simulink model "Strujni_nacin"  (R2023b)
settings: Solver=VariableStepAuto  StartTime=0.0  StopTime=stepp.sim_time  RelTol=1e-3
undefined symbols (not defined in the file or in its folder): ccm_m_op, G_sys_ccm, G_sys_dcm, G_Ubat_Ir_DCM, G_Ubat_Ir_full, G_Ubat_Ir_full_m, G_Ubat_Ir_nozero, G_Ubat_Ir_nozero_m, G_Ubat_Ir_red, G_Ubat_Ir_red_m, G_Ubat_Upv_DCM, G_Ubat_Upv_full, G_Ubat_Upv_full_m, G_Ubat_Upv_nozero, G_Ubat_Upv_nozero_m, G_Ubat_Upv_red, G_Ubat_Upv_red_m, G_UPV, G_Upv_IL, Ipv0, Ir, ro_ccm, ro_ccm_m, ro_dcm, stepp, Ubat0_ccm, Upv
settings Model: Creator=teo  LastModifiedBy=teo

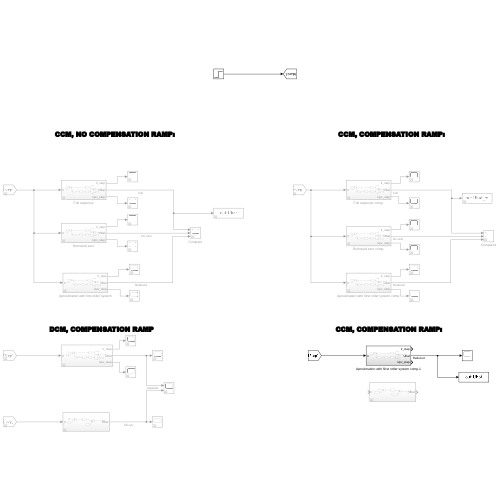
[thumbnail: Simulink's stored preview of the top-level diagram]
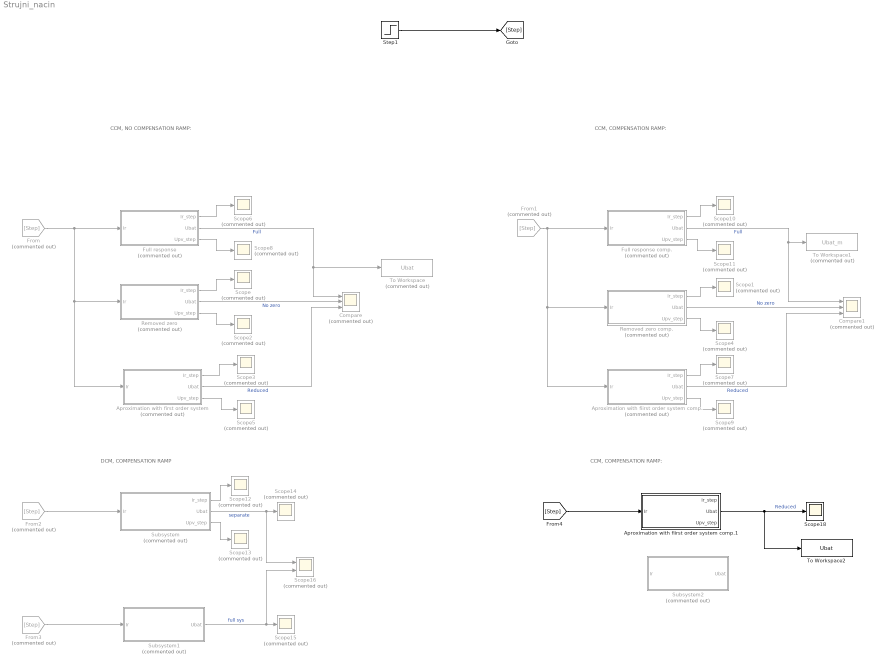
== system Strujni_nacin ==
  note: CCM, NO COMPENSATION RAMP:
  note: CCM, COMPENSATION RAMP:
  note: DCM, COMPENSATION RAMP
  note: CCM, COMPENSATION RAMP:
  Aproximation with fiirst order system comp. : Subsystem  Commented=on
  Aproximation with fiirst order system comp.1 : Subsystem
  Aproximation with first order system : Subsystem  Commented=on
  Compare : Scope  Commented=on  NumInputPorts=3
  Compare1 : Scope  Commented=on  NumInputPorts=3
  From{,1..3} (4 alike) : From  Commented=on  GotoTag=Step
  Full response : Subsystem  Commented=on
  Full response comp. : Subsystem  Commented=on
  Removed zero : Subsystem  Commented=on
  Removed zero comp. : Subsystem  Commented=on
  Scope{,1..15} (16 alike) : Scope  Commented=on
  Scope16 : Scope  Commented=on  NumInputPorts=2
  Scope18 : Scope
  Step1 : Step  Time=stepp.step_time  Before=stepp.ir01  After=stepp.ir02  SampleTime=0
  Subsystem : Subsystem  Commented=on
  Subsystem1 : Subsystem  Commented=on
  Subsystem2 : Subsystem  Commented=on
  To Workspace : ToWorkspace  Commented=on  VariableName=Ubat  SaveFormat=Timeseries  SampleTime=-1
  To Workspace1 : ToWorkspace  Commented=on  VariableName=Ubat_m  SaveFormat=Timeseries  SampleTime=-1
  To Workspace2 : ToWorkspace  VariableName=Ubat  SaveFormat=Timeseries  SampleTime=-1
  wires:
  Step1/1 -> [Step]
  From/1 -> Aproximation with first order system/1(Ir), Removed zero/1(Ir), Full response/1(Ir)
  Full response/1(Ir_step) -> Scope6/1
  Full response/3(Upv_step) -> Scope8/1
  Removed zero/1(Ir_step) -> Scope/1
  Removed zero/3(Upv_step) -> Scope2/1
  Aproximation with first order system/1(Ir_step) -> Scope3/1
  Aproximation with first order system/3(Upv_step) -> Scope5/1
  Removed zero/2(Ubat) -> Compare/2  "No zero"
  Full response/2(Ubat) -> To Workspace/1, Compare/1  "Full"
  Aproximation with first order system/2(Ubat) -> Compare/3  "Reduced"
  Full response comp./3(Upv_step) -> Scope11/1
  Full response comp./1(Ir_step) -> Scope10/1
  Removed zero comp./1(Ir_step) -> Scope1/1
  Removed zero comp./3(Upv_step) -> Scope4/1
  Aproximation with fiirst order system comp./1(Ir_step) -> Scope7/1
  Aproximation with fiirst order system comp./3(Upv_step) -> Scope9/1
  Full response comp./2(Ubat) -> To Workspace1/1, Compare1/1  "Full"
  Removed zero comp./2(Ubat) -> Compare1/2  "No zero"
  Aproximation with fiirst order system comp./2(Ubat) -> Compare1/3  "Reduced"
  From1/1 -> Aproximation with fiirst order system comp./1(Ir), Removed zero comp./1(Ir), Full response comp./1(Ir)
  From2/1 -> Subsystem/1(Ir)
  Subsystem/1(Ir_step) -> Scope12/1
  Subsystem/3(Upv_step) -> Scope13/1
  Subsystem/2(Ubat) -> Scope16/1, Scope14/1  "separate"
  From3/1 -> Subsystem1/1(Ir)
  Subsystem1/1(Ubat) -> Scope16/2, Scope15/1  "full sys"
  [Step] -> Aproximation with fiirst order system comp.1/1(Ir)
  Aproximation with fiirst order system comp.1/2(Ubat) -> To Workspace2/1, Scope18/1  "Reduced"

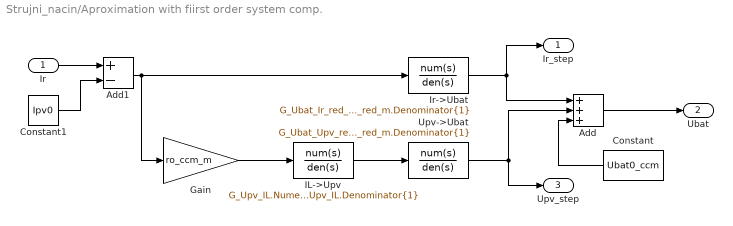
== system Strujni_nacin/Aproximation with fiirst order system comp. ==
  Ir : Inport
  Add : Sum  Inputs=+++
  Add1 : Sum  Inputs=+-
  Constant : Constant  Value=Ubat0_ccm
  Constant1 : Constant  Value=Ipv0
  Gain : Gain  Gain=ro_ccm_m
  IL->Upv : TransferFcn  Numerator=G_Upv_IL.Numerator{1}  Denominator=G_Upv_IL.Denominator{1}
  Ir->Ubat : TransferFcn  Numerator=G_Ubat_Ir_red_m.Numerator{1}  Denominator=G_Ubat_Ir_red_m.Denominator{1}
  Upv->Ubat : TransferFcn  Numerator=G_Ubat_Upv_red_m.Numerator{1}  Denominator=G_Ubat_Upv_red_m.Denominator{1}
  Ir_step : Outport
  Ubat : Outport  Port=2
  Upv_step : Outport  Port=3
  wires:
  Add1/1 -> Gain/1, Ir->Ubat/1
  Ir/1 -> Add1/1
  Gain/1 -> IL->Upv/1
  Constant1/1 -> Add1/2
  Upv->Ubat/1 -> Add/2, Upv_step/1
  Ir->Ubat/1 -> Add/1, Ir_step/1
  IL->Upv/1 -> Upv->Ubat/1
  Add/1 -> Ubat/1
  Constant/1 -> Add/3

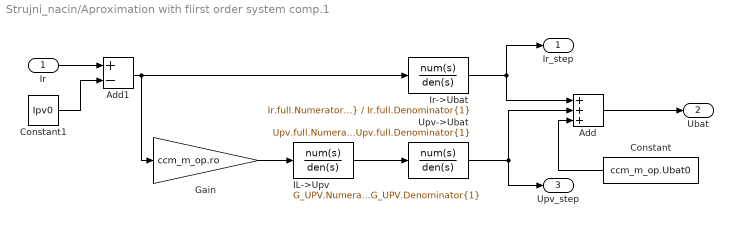
== system Strujni_nacin/Aproximation with fiirst order system comp.1 ==
  Ir : Inport
  Add : Sum  Inputs=+++
  Add1 : Sum  Inputs=+-
  Constant : Constant  Value=ccm_m_op.Ubat0
  Constant1 : Constant  Value=Ipv0
  Gain : Gain  Gain=ccm_m_op.ro
  IL->Upv : TransferFcn  Numerator=G_UPV.Numerator{1}  Denominator=G_UPV.Denominator{1}
  Ir->Ubat : TransferFcn  Numerator=Ir.full.Numerator{1}  Denominator=Ir.full.Denominator{1}
  Upv->Ubat : TransferFcn  Numerator=Upv.full.Numerator{1}  Denominator=Upv.full.Denominator{1}
  Ir_step : Outport
  Ubat : Outport  Port=2
  Upv_step : Outport  Port=3
  wires:
  Add1/1 -> Gain/1, Ir->Ubat/1
  Ir/1 -> Add1/1
  Gain/1 -> IL->Upv/1
  Constant1/1 -> Add1/2
  Upv->Ubat/1 -> Add/2, Upv_step/1
  Ir->Ubat/1 -> Add/1, Ir_step/1
  IL->Upv/1 -> Upv->Ubat/1
  Add/1 -> Ubat/1
  Constant/1 -> Add/3

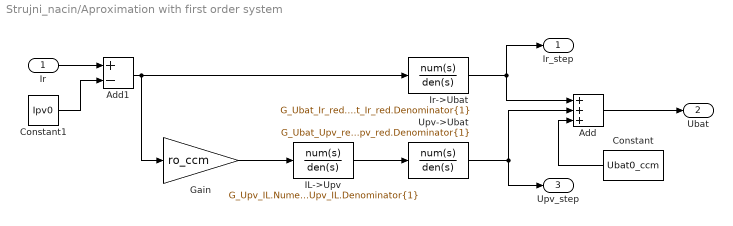
== system Strujni_nacin/Aproximation with first order system ==
  Ir : Inport
  Add : Sum  Inputs=+++
  Add1 : Sum  Inputs=+-
  Constant : Constant  Value=Ubat0_ccm
  Constant1 : Constant  Value=Ipv0
  Gain : Gain  Gain=ro_ccm
  IL->Upv : TransferFcn  Numerator=G_Upv_IL.Numerator{1}  Denominator=G_Upv_IL.Denominator{1}
  Ir->Ubat : TransferFcn  Numerator=G_Ubat_Ir_red.Numerator{1}  Denominator=G_Ubat_Ir_red.Denominator{1}
  Upv->Ubat : TransferFcn  Numerator=G_Ubat_Upv_red.Numerator{1}  Denominator=G_Ubat_Upv_red.Denominator{1}
  Ir_step : Outport
  Ubat : Outport  Port=2
  Upv_step : Outport  Port=3
  wires:
  Add1/1 -> Gain/1, Ir->Ubat/1
  Ir/1 -> Add1/1
  Gain/1 -> IL->Upv/1
  Constant1/1 -> Add1/2
  Upv->Ubat/1 -> Add/2, Upv_step/1
  Ir->Ubat/1 -> Add/1, Ir_step/1
  IL->Upv/1 -> Upv->Ubat/1
  Add/1 -> Ubat/1
  Constant/1 -> Add/3

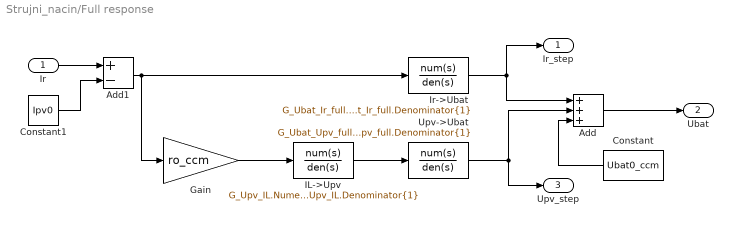
== system Strujni_nacin/Full response ==
  Ir : Inport
  Add : Sum  Inputs=+++
  Add1 : Sum  Inputs=+-
  Constant : Constant  Value=Ubat0_ccm
  Constant1 : Constant  Value=Ipv0
  Gain : Gain  Gain=ro_ccm
  IL->Upv : TransferFcn  Numerator=G_Upv_IL.Numerator{1}  Denominator=G_Upv_IL.Denominator{1}
  Ir->Ubat : TransferFcn  Numerator=G_Ubat_Ir_full.Numerator{1}  Denominator=G_Ubat_Ir_full.Denominator{1}
  Upv->Ubat : TransferFcn  Numerator=G_Ubat_Upv_full.Numerator{1}  Denominator=G_Ubat_Upv_full.Denominator{1}
  Ir_step : Outport
  Ubat : Outport  Port=2
  Upv_step : Outport  Port=3
  wires:
  Add1/1 -> Gain/1, Ir->Ubat/1
  Ir/1 -> Add1/1
  Gain/1 -> IL->Upv/1
  Constant1/1 -> Add1/2
  Upv->Ubat/1 -> Add/2, Upv_step/1
  Ir->Ubat/1 -> Add/1, Ir_step/1
  IL->Upv/1 -> Upv->Ubat/1
  Add/1 -> Ubat/1
  Constant/1 -> Add/3

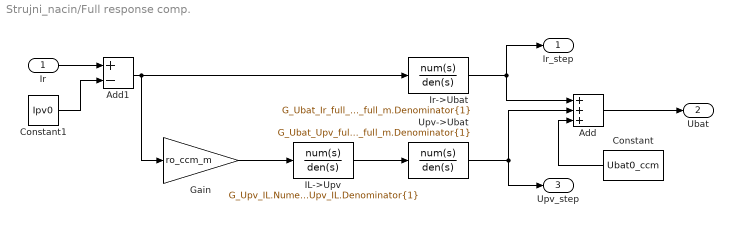
== system Strujni_nacin/Full response comp. ==
  Ir : Inport
  Add : Sum  Inputs=+++
  Add1 : Sum  Inputs=+-
  Constant : Constant  Value=Ubat0_ccm
  Constant1 : Constant  Value=Ipv0
  Gain : Gain  Gain=ro_ccm_m
  IL->Upv : TransferFcn  Numerator=G_Upv_IL.Numerator{1}  Denominator=G_Upv_IL.Denominator{1}
  Ir->Ubat : TransferFcn  Numerator=G_Ubat_Ir_full_m.Numerator{1}  Denominator=G_Ubat_Ir_full_m.Denominator{1}
  Upv->Ubat : TransferFcn  Numerator=G_Ubat_Upv_full_m.Numerator{1}  Denominator=G_Ubat_Upv_full_m.Denominator{1}
  Ir_step : Outport
  Ubat : Outport  Port=2
  Upv_step : Outport  Port=3
  wires:
  Add1/1 -> Gain/1, Ir->Ubat/1
  Ir/1 -> Add1/1
  Gain/1 -> IL->Upv/1
  Constant1/1 -> Add1/2
  Upv->Ubat/1 -> Add/2, Upv_step/1
  Ir->Ubat/1 -> Add/1, Ir_step/1
  IL->Upv/1 -> Upv->Ubat/1
  Add/1 -> Ubat/1
  Constant/1 -> Add/3

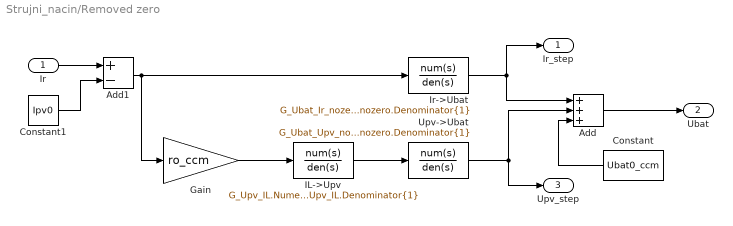
== system Strujni_nacin/Removed zero ==
  Ir : Inport
  Add : Sum  Inputs=+++
  Add1 : Sum  Inputs=+-
  Constant : Constant  Value=Ubat0_ccm
  Constant1 : Constant  Value=Ipv0
  Gain : Gain  Gain=ro_ccm
  IL->Upv : TransferFcn  Numerator=G_Upv_IL.Numerator{1}  Denominator=G_Upv_IL.Denominator{1}
  Ir->Ubat : TransferFcn  Numerator=G_Ubat_Ir_nozero.Numerator{1}  Denominator=G_Ubat_Ir_nozero.Denominator{1}
  Upv->Ubat : TransferFcn  Numerator=G_Ubat_Upv_nozero.Numerator{1}  Denominator=G_Ubat_Upv_nozero.Denominator{1}
  Ir_step : Outport
  Ubat : Outport  Port=2
  Upv_step : Outport  Port=3
  wires:
  Add1/1 -> Gain/1, Ir->Ubat/1
  Ir/1 -> Add1/1
  Gain/1 -> IL->Upv/1
  Constant1/1 -> Add1/2
  Upv->Ubat/1 -> Add/2, Upv_step/1
  Ir->Ubat/1 -> Add/1, Ir_step/1
  IL->Upv/1 -> Upv->Ubat/1
  Add/1 -> Ubat/1
  Constant/1 -> Add/3

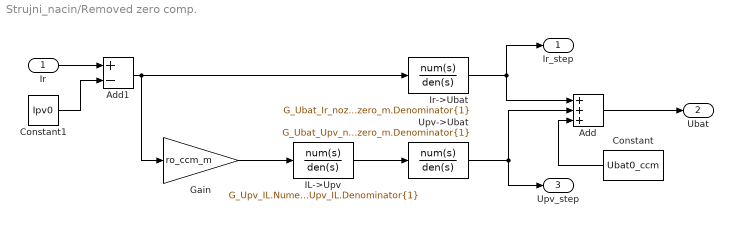
== system Strujni_nacin/Removed zero comp. ==
  Ir : Inport
  Add : Sum  Inputs=+++
  Add1 : Sum  Inputs=+-
  Constant : Constant  Value=Ubat0_ccm
  Constant1 : Constant  Value=Ipv0
  Gain : Gain  Gain=ro_ccm_m
  IL->Upv : TransferFcn  Numerator=G_Upv_IL.Numerator{1}  Denominator=G_Upv_IL.Denominator{1}
  Ir->Ubat : TransferFcn  Numerator=G_Ubat_Ir_nozero_m.Numerator{1}  Denominator=G_Ubat_Ir_nozero_m.Denominator{1}
  Upv->Ubat : TransferFcn  Numerator=G_Ubat_Upv_nozero_m.Numerator{1}  Denominator=G_Ubat_Upv_nozero_m.Denominator{1}
  Ir_step : Outport
  Ubat : Outport  Port=2
  Upv_step : Outport  Port=3
  wires:
  Add1/1 -> Gain/1, Ir->Ubat/1
  Ir/1 -> Add1/1
  Gain/1 -> IL->Upv/1
  Constant1/1 -> Add1/2
  Upv->Ubat/1 -> Add/2, Upv_step/1
  Ir->Ubat/1 -> Add/1, Ir_step/1
  IL->Upv/1 -> Upv->Ubat/1
  Add/1 -> Ubat/1
  Constant/1 -> Add/3

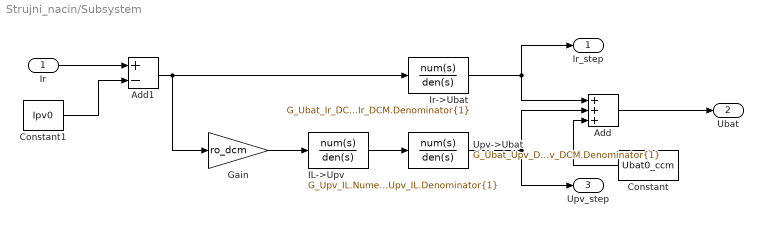
== system Strujni_nacin/Subsystem ==
  Ir : Inport
  Add : Sum  Inputs=+++
  Add1 : Sum  Inputs=+-
  Constant : Constant  Value=Ubat0_ccm
  Constant1 : Constant  Value=Ipv0
  Gain : Gain  Gain=ro_dcm
  IL->Upv : TransferFcn  Numerator=G_Upv_IL.Numerator{1}  Denominator=G_Upv_IL.Denominator{1}
  Ir->Ubat : TransferFcn  Numerator=G_Ubat_Ir_DCM.Numerator{1}  Denominator=G_Ubat_Ir_DCM.Denominator{1}
  Upv->Ubat : TransferFcn  Numerator=G_Ubat_Upv_DCM.Numerator{1}  Denominator=G_Ubat_Upv_DCM.Denominator{1}
  Ir_step : Outport
  Ubat : Outport  Port=2
  Upv_step : Outport  Port=3
  wires:
  IL->Upv/1 -> Upv->Ubat/1
  Constant/1 -> Add/3
  Upv->Ubat/1 -> Upv_step/1, Add/2
  Ir->Ubat/1 -> Ir_step/1, Add/1
  Add/1 -> Ubat/1
  Ir/1 -> Add1/1
  Constant1/1 -> Add1/2
  Add1/1 -> Gain/1, Ir->Ubat/1
  Gain/1 -> IL->Upv/1

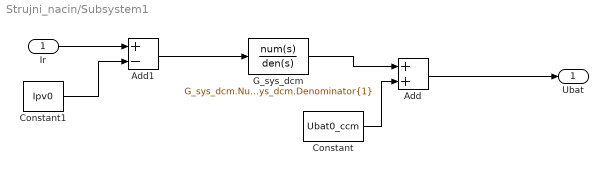
== system Strujni_nacin/Subsystem1 ==
  Ir : Inport
  Add : Sum
  Add1 : Sum  Inputs=+-
  Constant : Constant  Value=Ubat0_ccm
  Constant1 : Constant  Value=Ipv0
  G_sys_dcm : TransferFcn  Numerator=G_sys_dcm.Numerator{1}  Denominator=G_sys_dcm.Denominator{1}
  Ubat : Outport
  wires:
  G_sys_dcm/1 -> Add/1
  Constant/1 -> Add/2
  Add/1 -> Ubat/1
  Constant1/1 -> Add1/2
  Ir/1 -> Add1/1
  Add1/1 -> G_sys_dcm/1

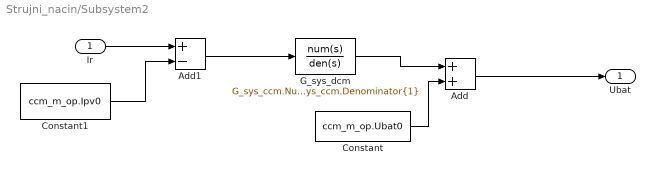
== system Strujni_nacin/Subsystem2 ==
  Ir : Inport
  Add : Sum
  Add1 : Sum  Inputs=+-
  Constant : Constant  Value=ccm_m_op.Ubat0
  Constant1 : Constant  Value=ccm_m_op.Ipv0
  G_sys_dcm : TransferFcn  Numerator=G_sys_ccm.Numerator{1}  Denominator=G_sys_ccm.Denominator{1}
  Ubat : Outport
  wires:
  G_sys_dcm/1 -> Add/1
  Constant/1 -> Add/2
  Add/1 -> Ubat/1
  Constant1/1 -> Add1/2
  Ir/1 -> Add1/1
  Add1/1 -> G_sys_dcm/1
